simulink model "luenberger_observer"  (R2019b)
settings: Solver=VariableStepAuto  StartTime=0.0  StopTime=10.0  RelTol=1e-3
undefined symbols (not defined in the file): A, Aob1, B, Bob1, C, C1, Cob1, Dob1
settings Model: Creator=Anubhav Paras  LastModifiedBy=Anubhav Paras

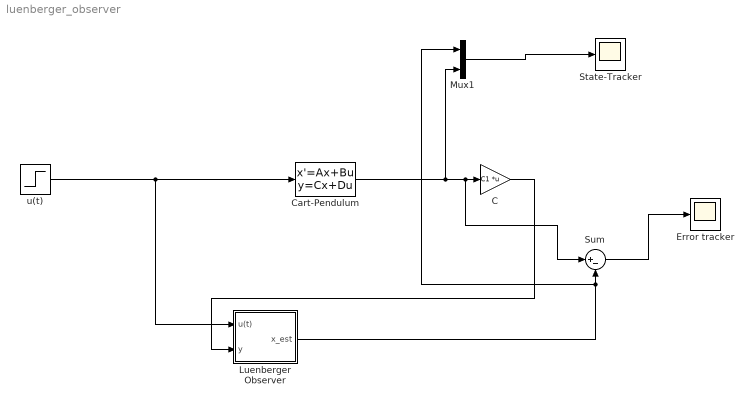
== system luenberger_observer ==
  " Luenberger Observer" : Subsystem
  C : Gain  Gain=C1  Multiplication=Matrix(K*u)
  "Cart-Pendulum " : StateSpace  A=A  B=B  C=C  D=zeros(6,1)  InitialCondition=0
  Error tracker : Scope
  Mux1 : Mux  Inputs=2
  State-Tracker : Scope
  Sum : Sum  Inputs=|+-
  u(t) : Step  SampleTime=0
  wires:
  u(t)/1 -> " Luenberger Observer"/1(u(t)), "Cart-Pendulum "/1
  Sum/1 -> Error tracker/1
  "Cart-Pendulum "/1 -> Mux1/2, Sum/1, C/1
  Mux1/1 -> State-Tracker/1
  " Luenberger Observer"/1(x_est) -> Mux1/1, Sum/2
  C/1 -> " Luenberger Observer"/2(y)

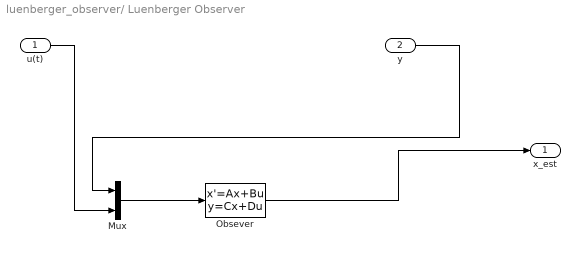
== system luenberger_observer/ Luenberger Observer ==
  u(t) : Inport
  y : Inport  Port=2
  Mux : Mux  Inputs=2
  "Obsever " : StateSpace  A=Aob1  B=Bob1  C=Cob1  D=Dob1  InitialCondition=0
  x_est : Outport
  wires:
  Mux/1 -> "Obsever "/1
  "Obsever "/1 -> x_est/1
  y/1 -> Mux/1
  u(t)/1 -> Mux/2
